simulink model "11lab"  (R2024a)
settings: Solver=VariableStepAuto  StartTime=0.0  StopTime=60.0  RelTol=1e-3
undefined symbols (not defined in the file): entity, m, n, sumTimer
libraries: simulink x2
settings Model: Creator=94410  LastModifiedBy=94410

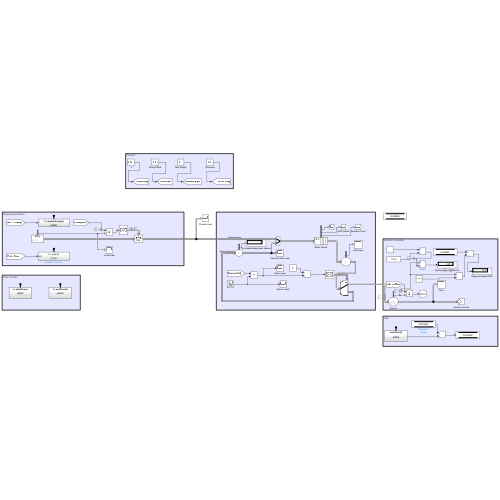
[thumbnail: Simulink's stored preview of the top-level diagram]
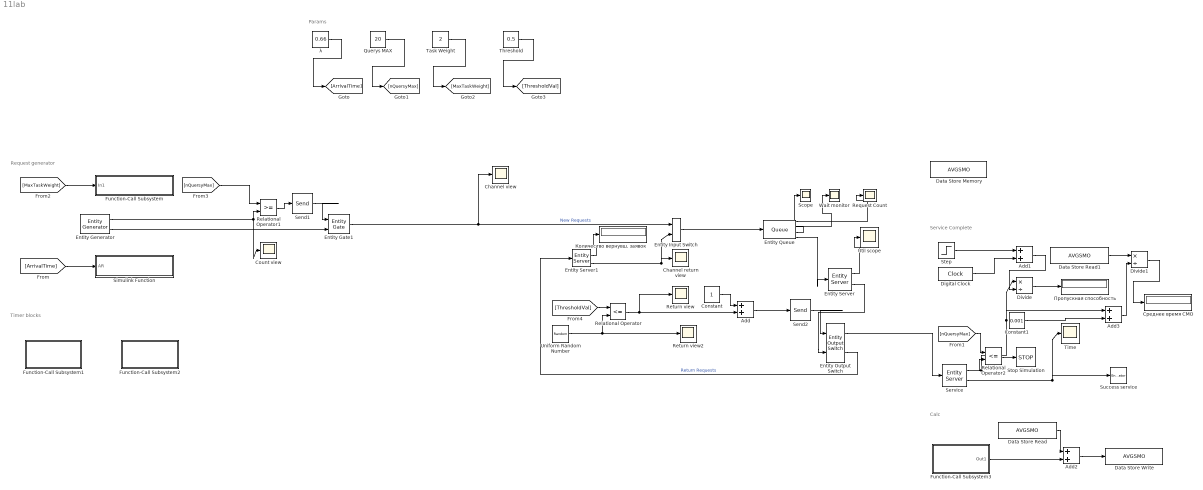
== system 11lab ==
  note: Calc
  note: Timer blocks
  note: Request generator
  note: Params
  note: Service Complete
  " Querys MAX" : Constant  Value=20  SampleTime=-1
  " λ" : Constant  Value=0.66  SampleTime=-1
  Add{,1..3} (4 alike) : Sum
  Channel return view : Scope
  Channel view : Scope
  Constant : Constant  SampleTime=-1
  Constant1 : Constant  Value=0.001
  Count view : Scope
  Data Store Memory : DataStoreMemory  DataStoreName=AVGSMO  WriteAfterWriteMsg=warning  InitialValue=0.1  ShowAdditionalParam=off
  Data Store Read : DataStoreRead  DataStoreName=AVGSMO  IndexOptions=Index vector (dialog)  Indices=1  OutputSizes=1
  Data Store Read1 : DataStoreRead  DataStoreName=AVGSMO  IndexOptions=Index vector (dialog)  Indices=1  OutputSizes=1
  Data Store Write : DataStoreWrite  DataStoreName=AVGSMO  IndexOptions=Index vector (dialog)  Indices=1  OutputSizes=1
  Digital Clock : DigitalClock
  Divide : Product  Inputs=*/
  Divide1 : Product  Inputs=*/
  Entity Input Switch : EntityInputSwitch  InputPortMessageModes=m,m  OutputPortMessageModes=m
  Entity Output Switch : EntityOutputSwitch  InputPortMessageModes=m,m  OutputPortMessageModes=m,m  SwitchingCriterion=From control port  SwitchAttributeName=Attribute1
      settings: InputPortMap=u0,u1
  Entity Gate1 : EntityGate  InputPortMessageModes=m,m  OutputPortMessageModes=m  OperatingMode=Release gate  OpenGateAtSimulationStart=on
  Entity Generator : EntityGenerator  OutputPortMessageModes=n,m  TimeSource=MATLAB action  Period=5  IntergenerationTimeAction=dt = expAT();  GenerateAction=entity.SMOTime = startTimer();  AttributeName=entity|ServiceTime|SMOTime  AttributeInitialValue=0|1|1  NumberEntitiesDeparted=on  EntityType=Structured  EntityTypeName=Entity
      settings: OutputPortMap=o0,o3
  Entity Queue : Queue  InputPortMessageModes=m  OutputPortMessageModes=n,n,n,m  Capacity=inf  PrioritySource=entitySys.priority  SortingDirection=Descending  NumberEntitiesInBlock=on  AverageWait=on  AverageQueueLength=on
      settings: OutputPortMap=o1,o2,o3,o5
  Entity Server : EntityServer  InputPortMessageModes=m  OutputPortMessageModes=n,m  Capacity=1  ServiceTimeSource=Attribute  ServiceTimeAction=dt = entitySys.priority;  Utilization=on
      settings: OutputPortMap=o5,o9
  Entity Server1 : EntityServer  InputPortMessageModes=m  OutputPortMessageModes=n,m  Capacity=1  ServiceTimeValue=0  NumberEntitiesDeparted=on
      settings: OutputPortMap=o0,o9
  Function-Call Subsystem : Subsystem  TreatAsAtomicUnit=on
  Function-Call Subsystem1 : Subsystem  TreatAsAtomicUnit=on
  Function-Call Subsystem2 : Subsystem  TreatAsAtomicUnit=on
  Function-Call Subsystem3 : Subsystem  TreatAsAtomicUnit=on
  Relational Operator : RelationalOperator  Operator=<=  OutDataTypeStr=boolean  RndMeth=Simplest  InputSameDT=off
  Relational Operator1 : RelationalOperator  OutDataTypeStr=boolean  RndMeth=Simplest  InputSameDT=off
  Relational Operator2 : RelationalOperator  Operator=<=  OutDataTypeStr=boolean  RndMeth=Simplest  InputSameDT=off
  Request Count : Scope
  Return view : Scope
  Return view2 : Scope
  Scope : Scope
  Send1 : Send  OutputPortMessageModes=m
  Send2 : Send  OutputPortMessageModes=m
  Service : EntityServer  InputPortMessageModes=m  OutputPortMessageModes=n,m  Capacity=1  ServiceTimeValue=0  EntryAction=entity.SMOTime = endTimer(entity.SMOTime);  ServiceCompleteAction=sumTimer(entity.SMOTime)  NumberEntitiesDeparted=on
      settings: OutputPortMap=o0,o9
  Simulink Function : Subsystem  TreatAsAtomicUnit=on
  Step : Step  Before=1  SampleTime=0
  Stop Simulation : Stop
  Success service : EntityTerminator  InputPortMessageModes=m
  Task Weight : Constant  Value=2  SampleTime=-1
  Threshold : Constant  Value=0.5  SampleTime=-1
  Time : Scope
  Uniform Random Number : UniformRandomNumber  Minimum=0  Seed=3748724  SampleTime=0  VectorParams1D=off
  Util scope : Scope
  Wait monitor : Scope
  Количество вернувш. заявок : Display
  Пропускная способность : Display
  Среднее время СМО : Display
  wires:
  Relational Operator/1 -> Add/2, Return view/1
  Entity Input Switch/1 -> Entity Queue/1
  Entity Server/1 -> Util scope/1
  Relational Operator1/1 -> Send1/1
  Send2/1 -> Entity Output Switch/1
  Entity Generator/2 -> Entity Gate1/2
  Entity Output Switch/2 -> Entity Server1/1  "Return Requests"
  Uniform Random Number/1 -> Relational Operator/2, Return view2/1
  [nQuersyMax] -> Relational Operator1/1
  [ThresholdVal] -> Relational Operator/1
  Send1/1 -> Entity Gate1/1
  Entity Server/2 -> Entity Output Switch/2
  Entity Gate1/1 -> Channel view/1, Entity Input Switch/1  "New Requests"
  Task Weight/1 -> [MaxTaskWeight]
  " λ"/1 -> [ArrivalTime]
  [ArrivalTime] -> Simulink Function/1(AR)
  [MaxTaskWeight] -> Function-Call Subsystem/1(In1)
  Entity Queue/2 -> Wait monitor/1
  " Querys MAX"/1 -> [nQuersyMax]
  Entity Generator/1 -> Count view/1, Relational Operator1/2
  Threshold/1 -> [ThresholdVal]
  Entity Queue/4 -> Entity Server/1
  Entity Queue/1 -> Request Count/1
  Entity Server1/1 -> Количество вернувш. заявок/1
  Entity Server1/2 -> Channel return view/1, Entity Input Switch/2
  Entity Output Switch/1 -> Service/1
  Service/1 -> Divide/1, Add3/1, Relational Operator2/2
  [nQuersyMax] -> Relational Operator2/1
  Relational Operator2/1 -> Stop Simulation/1
  Entity Queue/3 -> Scope/1
  Add/1 -> Send2/1
  Constant/1 -> Add/1
  Step/1 -> Add1/1
  Digital Clock/1 -> Add1/2
  Add1/1 -> Divide/2
  Divide/1 -> Пропускная способность/1
  Service/2 -> Success service/1, Time/1
  Data Store Read/1 -> Add2/1
  Add2/1 -> Data Store Write/1
  Data Store Read1/1 -> Divide1/1
  Divide1/1 -> Среднее время СМО/1
  Function-Call Subsystem3/1(Out1) -> Add2/2
  Constant1/1 -> Add3/2
  Add3/1 -> Divide1/2

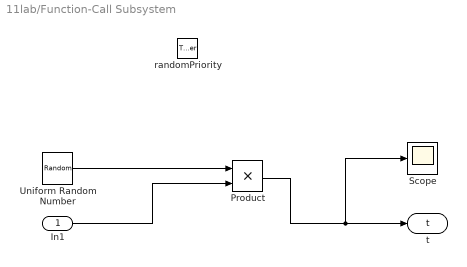
== system 11lab/Function-Call Subsystem ==
  In1 : Inport
  randomPriority : TriggerPort  TriggerType=function-call  IsSimulinkFunction=on  FunctionName=randomPriority  VariantControl=(inherit)
  Product : Product
  Scope : Scope
  Uniform Random Number : UniformRandomNumber  Minimum=0  Seed=12345  VectorParams1D=off
  t : ArgOut  DisableCoverage=on  ArgumentName=t
  wires:
  In1/1 -> Product/2
  Uniform Random Number/1 -> Product/1
  Product/1 -> Scope/1, t/1

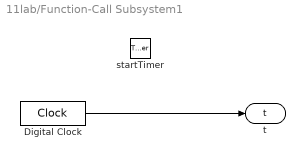
== system 11lab/Function-Call Subsystem1 ==
  startTimer : TriggerPort  TriggerType=function-call  IsSimulinkFunction=on  FunctionName=startTimer  VariantControl=(inherit)
  Digital Clock : DigitalClock  SampleTime=-1
  t : ArgOut  DisableCoverage=on  ArgumentName=t
  wires:
  Digital Clock/1 -> t/1

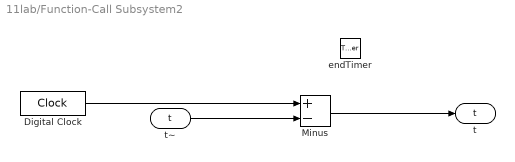
== system 11lab/Function-Call Subsystem2 ==
  endTimer : TriggerPort  TriggerType=function-call  IsSimulinkFunction=on  FunctionName=endTimer  VariantControl=(inherit)
  Digital Clock : DigitalClock  SampleTime=-1
  Minus : Sum  Inputs=+-
  t~ : ArgIn  ArgumentName=t
  t : ArgOut  DisableCoverage=on  ArgumentName=t
  wires:
  Minus/1 -> t/1
  t~/1 -> Minus/2
  Digital Clock/1 -> Minus/1

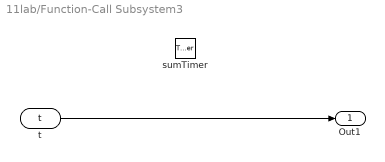
== system 11lab/Function-Call Subsystem3 ==
  sumTimer : TriggerPort  TriggerType=function-call  IsSimulinkFunction=on  FunctionName=sumTimer  VariantControl=(inherit)
  t : ArgIn  ArgumentName=t
  Out1 : Outport
  wires:
  t/1 -> Out1/1

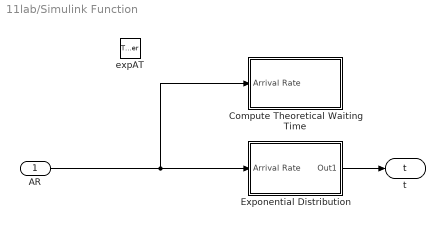
== system 11lab/Simulink Function ==
  AR : Inport
  expAT : TriggerPort  TriggerType=function-call  IsSimulinkFunction=on  FunctionName=expAT  VariantControl=Variant
  Compute Theoretical Waiting Time : Subsystem
  Exponential Distribution : Subsystem
  t : ArgOut  DisableCoverage=on  ArgumentName=t
  wires:
  AR/1 -> Compute Theoretical Waiting Time/1(Arrival Rate), Exponential Distribution/1(Arrival Rate)
  Exponential Distribution/1(Out1) -> t/1

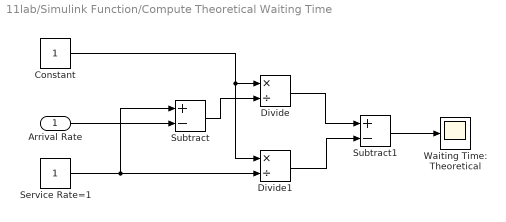
== system 11lab/Simulink Function/Compute Theoretical Waiting Time ==
  Arrival Rate : Inport
  Constant : Constant
  Divide : Product  Inputs=*/
  Divide1 : Product  Inputs=*/
  Service Rate=1 : Constant
  Subtract : Sum  Inputs=+-
  Subtract1 : Sum  Inputs=+-
  Waiting Time: Theoretical : Scope
  wires:
  Arrival Rate/1 -> Subtract/2
  Subtract1/1 -> Waiting Time: Theoretical/1
  Divide1/1 -> Subtract1/2
  Divide/1 -> Subtract1/1
  Subtract/1 -> Divide/2
  Constant/1 -> Divide1/1, Divide/1
  Service Rate=1/1 -> Subtract/1, Divide1/2

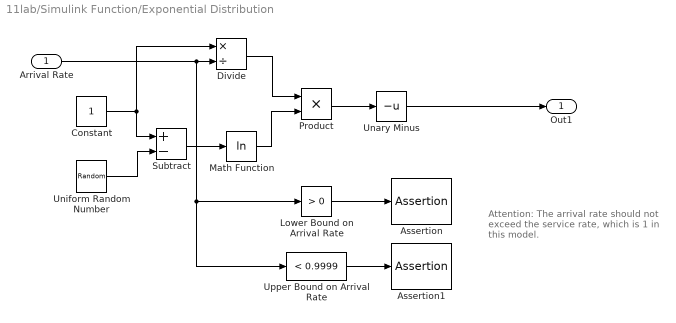
== system 11lab/Simulink Function/Exponential Distribution ==
  note: Attention: The arrival rate
      | should not exceed the service
      | rate, which is 1 in this model.
  Arrival Rate : Inport
  Assertion : Assertion
  Assertion1 : Assertion
  Constant : Constant
  Divide : Product  Inputs=*/
  Lower Bound on Arrival Rate : simulink/Logic and Bit Operations/Compare To Constant  relop=>  const=0  OutDataTypeStr=uint8  ZeroCross=off
  Math Function : Math  Operator=log  SignedPower=on
  Product : Product  RndMeth=Zero
  Subtract : Sum  Inputs=+-
  Unary Minus : UnaryMinus
  Uniform Random Number : UniformRandomNumber  Minimum=0  Seed=12345
  "Upper Bound on Arrival Rate " : simulink/Logic and Bit Operations/Compare To Constant  relop=<  const=0.9999  OutDataTypeStr=uint8  ZeroCross=off
  Out1 : Outport
  wires:
  Arrival Rate/1 -> Divide/2, Lower Bound on Arrival Rate/1, "Upper Bound on Arrival Rate "/1
  Unary Minus/1 -> Out1/1
  Product/1 -> Unary Minus/1
  Math Function/1 -> Product/2
  Divide/1 -> Product/1
  Constant/1 -> Divide/1, Subtract/1
  Uniform Random Number/1 -> Subtract/2
  Lower Bound on Arrival Rate/1 -> Assertion/1
  "Upper Bound on Arrival Rate "/1 -> Assertion1/1
  Subtract/1 -> Math Function/1
